simulink model "trajectory_planning_tests"  (R2022a)
settings: Solver=VariableStepAuto  StartTime=0  StopTime=sim_time  FixedStep=0.01  RelTol=1e-3
InitFcn:
  | trajectory_planning
values from neighbouring files (symbols this model uses):
  A = zeros(6)    [find_path_coeffs.m]    (also in getLateralDynamics.m = [0 1 vx 0)
  B = [0; -b1; 0; -b2]    [getLateralDynamics.m]
  C = [1 0 d 0]    [lat_sim_parameters.m]
  CfReal = alpha*Cf    (= 12000)    [lat_sim_parameters.m]
  CrReal = beta*Cr    (= 11000)    [lat_sim_parameters.m]
  Iz = 2875    [acc_sim_parameters.m]    (also in lat_sim_parameters.m = 4000; tuneLateralController.m = 4000)
  Klat = place(A, B, poles)    [lat_sim_parameters.m]    (also in tuneLateralController.m)
  lf = 1.2    [acc_sim_parameters.m]    (also in lat_sim_parameters.m = 3; tuneLateralController.m = 3)
  lr = 1.6    [acc_sim_parameters.m]    (also in lat_sim_parameters.m = 2; tuneLateralController.m = 2)
  m = 1575    [acc_sim_parameters.m]    (also in lat_sim_parameters.m = 2000; tuneLateralController.m = 2000)
  start_time = 1    [computeLateralReferenceTrajectory.m]    (also in trajectory_planning.m)
undefined symbols (not defined in the file or in its folder): vxBar
libraries: autolibshared x1
settings Model: Creator=Fernando VM  LastModifiedBy=fvall
settings SolverCC: AlgebraicLoopSolver=TrustRegion
settings DataIOCC: ExternalInput=[dt, da, dd]  ReturnWorkspaceOutputs=off
settings DebuggingCC: UnconnectedInputMsg=warning  UnconnectedOutputMsg=warning  UnconnectedLineMsg=warning  SFMachineParentedDataDiag=warning  ArithmeticOperatorsInVariantConditions=warning
settings SFSimCC: CustomCodeUndefinedFunction=UseInterfaceOnly

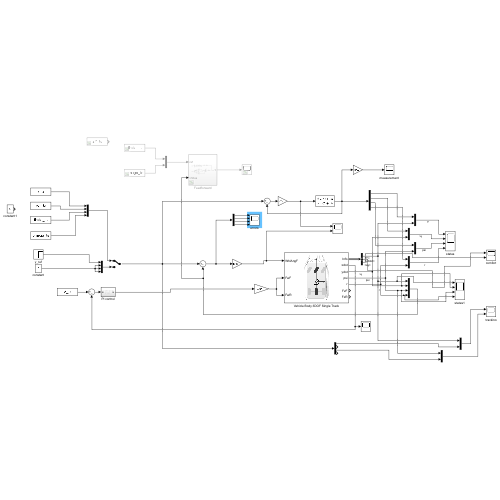
[thumbnail: Simulink's stored preview of the top-level diagram]
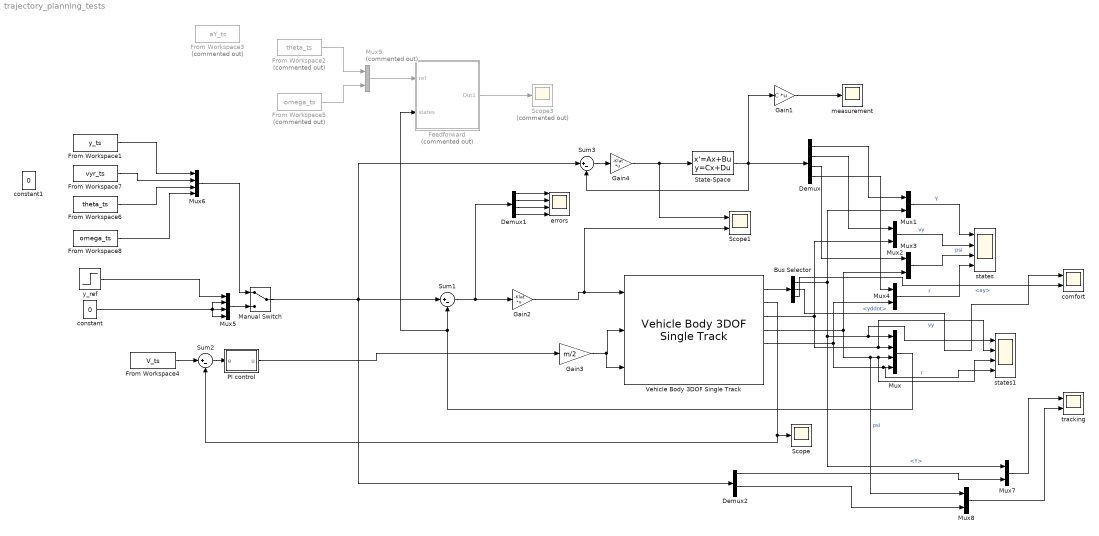
== system trajectory_planning_tests ==
  Bus Selector : BusSelector  OutputSignals=InertFrm.Cg.Disp.Y,BdyFrm.Cg.Acc.yddot,BdyFrm.Cg.Acc.ay
  Demux : Demux
  Demux1 : Demux
  Demux2 : Demux
  Feedforward : Subsystem  Commented=on
  From Workspace1 : FromWorkspace  VariableName=y_ts
  From Workspace2 : FromWorkspace  Commented=on  VariableName=theta_ts
  From Workspace3 : FromWorkspace  Commented=on  VariableName=aY_ts
  From Workspace4 : FromWorkspace  VariableName=V_ts
  From Workspace5 : FromWorkspace  Commented=on  VariableName=omega_ts
  From Workspace6 : FromWorkspace  VariableName=theta_ts
  From Workspace7 : FromWorkspace  VariableName=vyr_ts
  From Workspace8 : FromWorkspace  VariableName=omega_ts
  Gain1 : Gain  Gain=C  Multiplication=Matrix(K*u)
  Gain2 : Gain  Gain=-Klat  Multiplication=Matrix(K*u)
  Gain3 : Gain  Gain=m/2
  Gain4 : Gain  Gain=-Klat  Multiplication=Matrix(K*u)
  Manual Switch : ManualSwitch
  Mux : Mux
  Mux{1..4,7..8} (6 alike) : Mux  Inputs=2
  Mux5 : Mux
  Mux6 : Mux
  Mux9 : Mux  Commented=on  Inputs=2
  PI control : Subsystem
  Scope : Scope
  Scope1 : Scope  NumInputPorts=2
  Scope3 : Scope  Commented=on
  State-Space : StateSpace  A=A  B=B  C=eye(4)  D=zeros(4,1)  InitialCondition=[0; 0 ; 0; 0]
  Sum1 : Sum  Inputs=|+-
  Sum2 : Sum  Inputs=|+-
  Sum3 : Sum  Inputs=|+-
  Vehicle Body 3DOF Single Track : autolibshared/Vehicle Body 3DOF Single Track  trackMode=Single (bicycle)  inputMode=External longitudinal forces  frontSteerMode=on  rearSteerMode=off  windMode=off  muMode=off  extFMode=off  extMMode=off  htchFMode=off  htchMMode=off  extXo=off  extpsio=off  extxdoto=off  extro=off  extYo=off  extTamb=off  extydoto=off  aMode=2  NF=2  NR=2  m=m  a=lf  b=lr  h=0.35  dh=1  hh=0.2  X_o=0  xdot_o=vx0  CalphaMode=off  sigmaMode=on  d=0  hl=0  w=[1.4,1.4]  Cy_f=CfReal  Cy_r=CrReal  sigma_f=.1  sigma_r=.1  alpha_f_brk=[-.1 .1]  Cy_f_data=[-9e3 9e3]  alpha_r_brk=[-.1 .1]  Cy_r_data=[-9e3 9e3]  Y_o=0  ydot_o=0  Izz=Iz  psi_o=0  r_o=0  Af=2  Cd=.3  Cl=.1  Cpm=.1  beta_w=[0:0.01:0.3]  Cs=[0:0.03:0.9]  Cym=[0:0.01:0.3]  Pabs=101325  Tair=273  g=9.81  mu=1  xdot_tol=.01  Fznom=5000  Fxtire_sat=7e4  Fytire_sat=7e4  longOff=0  latOff=0  vertOff=0  wrapAng=off
      settings: SourceProductBaseCode=PW,DR,MT,VE
  comfort : Scope  NumInputPorts=2
  constant : Constant  Value=0
  constant1 : Constant  Value=0
  errors : Scope  NumInputPorts=4
  measurement : Scope
  states : Scope  NumInputPorts=4
  states1 : Scope  NumInputPorts=4
  tracking : Scope  NumInputPorts=2
  y_ref : Step  Time=start_time  After=4  SampleTime=0
  wires:
  Gain1/1 -> measurement/1
  Gain4/1 -> Scope1/1, State-Space/1
  State-Space/1 -> Sum3/2, Gain1/1, Demux/1
  Demux/1 -> Mux1/1
  Sum1/1 -> Demux1/1, Gain2/1
  Feedforward/1(Out1) -> Scope3/1
  Vehicle Body 3DOF Single Track/1 -> Bus Selector/1
  Bus Selector/1 -> Mux7/1, states1/1, Mux/1, Mux1/2  "<Y>"
  Vehicle Body 3DOF Single Track/3 -> states1/2, Mux/2, Mux2/2  "vy"
  Vehicle Body 3DOF Single Track/4 -> Mux8/1, states1/3, Mux/3, Mux3/2  "psi"
  Vehicle Body 3DOF Single Track/5 -> states1/4, Mux/4, Mux4/2  "r"
  Mux1/1 -> states/1  "Y"
  Demux/2 -> Mux2/1
  Demux/3 -> Mux3/1
  Demux/4 -> Mux4/1
  Mux2/1 -> states/2  "vy"
  Mux3/1 -> states/3  "psi"
  Mux4/1 -> states/4  "r"
  Gain3/1 -> Vehicle Body 3DOF Single Track/3, Vehicle Body 3DOF Single Track/2
  From Workspace4/1 -> Sum2/1
  Vehicle Body 3DOF Single Track/2 -> Sum2/2, Scope/1
  Bus Selector/2 -> comfort/1  "<yddot>"
  Sum2/1 -> PI control/1(e)
  PI control/1(u) -> Gain3/1
  constant/1 -> Mux5/4, Mux5/2, Mux5/3
  y_ref/1 -> Mux5/1
  Sum3/1 -> Gain4/1
  Demux1/1 -> errors/1
  Demux1/2 -> errors/2
  Demux1/3 -> errors/3
  Demux1/4 -> errors/4
  Mux5/1 -> Manual Switch/2
  Mux6/1 -> Manual Switch/1
  Demux2/1 -> Mux7/2
  Mux7/1 -> tracking/1
  Demux2/3 -> Mux8/2
  Mux8/1 -> tracking/2
  From Workspace7/1 -> Mux6/2
  Bus Selector/3 -> comfort/2  "<ay>"
  Gain2/1 -> Scope1/2, Vehicle Body 3DOF Single Track/1
  Manual Switch/1 -> Sum1/1, Demux2/1, Sum3/1
  Mux/1 -> Feedforward/2(states), Sum1/2
  Mux9/1 -> Feedforward/1(ref)
  From Workspace2/1 -> Mux9/1
  From Workspace5/1 -> Mux9/2
  From Workspace1/1 -> Mux6/1
  From Workspace6/1 -> Mux6/3
  From Workspace8/1 -> Mux6/4

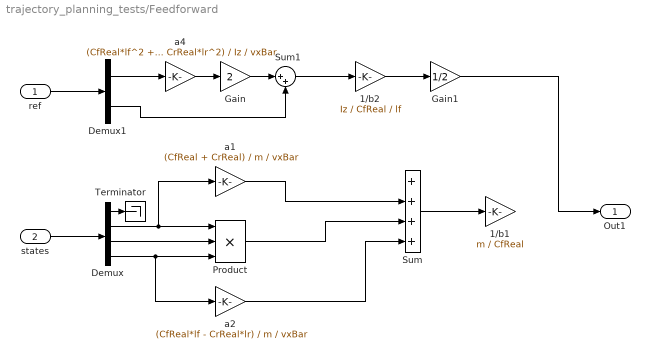
== system trajectory_planning_tests/Feedforward ==
  ref : Inport
  states : Inport  Port=2
  1/b1 : Gain  Gain=m / CfReal
  1/b2 : Gain  Gain=Iz / CfReal / lf
  Demux : Demux
  Demux1 : Demux  Outputs=2
  Gain : Gain  Gain=2
  Gain1 : Gain  Gain=1/2
  Product : Product  Inputs=3
  Sum : Sum  Inputs=++++
  Sum1 : Sum  Inputs=|++
  Terminator : Terminator
  a1 : Gain  Gain=(CfReal + CrReal) / m / vxBar
  a2 : Gain  Gain=(CfReal*lf - CrReal*lr) / m / vxBar
  a4 : Gain  Gain=(CfReal*lf^2 + CrReal*lr^2) / Iz / vxBar
  Out1 : Outport
  wires:
  ref/1 -> Demux1/1
  states/1 -> Demux/1
  Demux/2 -> Product/1, a1/1
  Demux/4 -> Product/3, a2/1
  Demux/3 -> Product/2
  a1/1 -> Sum/2
  Product/1 -> Sum/3
  a2/1 -> Sum/4
  Sum/1 -> 1/b1/1
  1/b2/1 -> Gain1/1
  Demux/1 -> Terminator/1
  Demux1/1 -> a4/1
  a4/1 -> Gain/1
  Demux1/2 -> Sum1/2
  Sum1/1 -> 1/b2/1
  Gain/1 -> Sum1/1
  Gain1/1 -> Out1/1

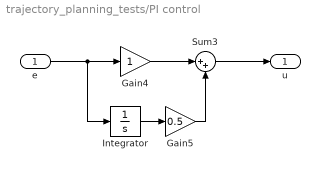
== system trajectory_planning_tests/PI control ==
  e : Inport
  Gain4 : Gain
  Gain5 : Gain  Gain=0.5
  Integrator : Integrator
  Sum3 : Sum  Inputs=|++
  u : Outport  VectorParamsAs1DForOutWhenUnconnected=off
  wires:
  e/1 -> Gain4/1, Integrator/1
  Sum3/1 -> u/1
  Gain4/1 -> Sum3/1
  Integrator/1 -> Gain5/1
  Gain5/1 -> Sum3/2
